simulink model "question10_2018b"  (R2018b)
settings: Solver=VariableStepAuto  StartTime=0.0  StopTime=100  RelTol=1e-3
values from neighbouring files (symbols this model uses):
  A = [ 0 1 0 0 ... (first row only)    [Alt_Industrial_plant.m]    (also in IndustrialPlant.m; ObserverExample.m = [0 1 0; 980  0  -2.8; 0 0 -100]; OldProject.m = [0 1 0 0 ;-491 0 -282.45 0; 0 0 0 1;1488 0 885.65 0]; observerWorkingExample.m = [0, 0, 1, 0)
  Ad = sys_d.a    [Alt_Industrial_plant.m]    (also in observerWorkingExample.m)
  B = [0; 1/Jd; 0; 0]    [Alt_Industrial_plant.m]    (also in IndustrialPlant.m; ObserverExample.m = [ 0; 0; 100]; OldProject.m = [0;82.33;0;-235.29]; observerWorkingExample.m = [0; 0; 1/mc; 1/(L*mc)])
  Bd = sys_d.b    [Alt_Industrial_plant.m]    (also in observerWorkingExample.m)
  Cd = sys_d.c    [Alt_Industrial_plant.m]    (also in observerWorkingExample.m)
  K = acker(A,B,des_poles)    [Alt_Industrial_plant.m]    (also in ObserverExample.m = place(A,B,[p1 p2 p3]); OldProject.m = place(A,B,Pole_fb); observerWorkingExample.m)
  K_d = acker(Ad,Bd,des_poles_d)    [Alt_Industrial_plant.m]    (also in observerWorkingExample.m)
  Ob = place(A',C,obs_poles)    [Alt_Industrial_plant.m]    (also in observerWorkingExample.m = acker(Ad',Cd',des_poles_d))
  Ob_d = acker(Ad',Cd',des_poles_d)    [Alt_Industrial_plant.m]
  Ts = 0.1    [Alt_Industrial_plant.m]    (also in observerWorkingExample.m)
  x0 = [0;15*pi/180;0;0]    [Alt_Industrial_plant.m]    (also in ObserverExample.m = [0.01 0.5 -5]; observerWorkingExample.m = [0;5*pi/180;0;0])
settings Model: Creator=Yaipiti  LastModifiedBy=Dimitri
settings DataIOCC: ReturnWorkspaceOutputs=on

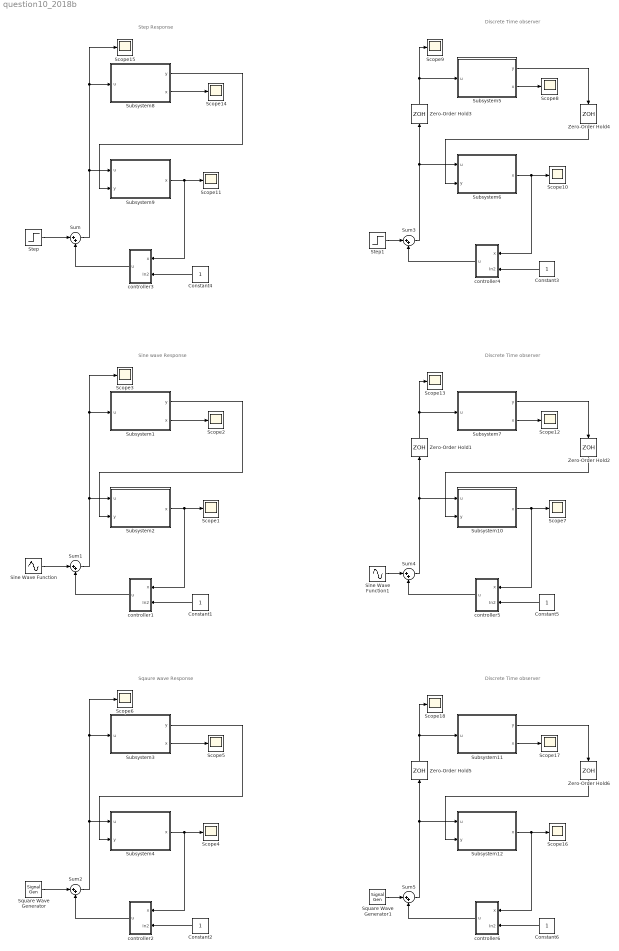
== system question10_2018b ==
  note: Step Response
  note: Sine wave Response
  note: Sqaure wave Response
  note: Discrete Time observer
  note: Discrete Time observer
  note: Discrete Time observer
  Constant{1..6} (6 alike) : Constant
  Scope{1..18} (18 alike) : Scope
  Sine Wave Function : Sin  Amplitude=2  Frequency=0.1  SampleTime=0
  Sine Wave Function1 : Sin  Amplitude=2  Frequency=0.1  SampleTime=0
  Square Wave Generator : SignalGenerator  WaveForm=square  Amplitude=5  Units=rad/sec
  Square Wave Generator1 : SignalGenerator  WaveForm=square  Amplitude=5  Units=rad/sec
  Step : Step  Time=2  SampleTime=0
  Step1 : Step  Time=2  SampleTime=0
  Subsystem1 : Subsystem
  Subsystem10 : Subsystem
  Subsystem11 : Subsystem
  Subsystem12 : Subsystem
  Subsystem2 : Subsystem
  Subsystem3 : Subsystem
  Subsystem4 : Subsystem
  Subsystem5 : Subsystem
  Subsystem6 : Subsystem
  Subsystem7 : Subsystem
  Subsystem8 : Subsystem
  Subsystem9 : Subsystem
  Sum{,1..5} (6 alike) : Sum  Inputs=|++
  Zero-Order Hold{1..6} (6 alike) : ZeroOrderHold  SampleTime=Ts
  controller1 : Subsystem
  controller2 : Subsystem
  controller3 : Subsystem
  controller4 : Subsystem
  controller5 : Subsystem
  controller6 : Subsystem
  wires:
  Constant4/1 -> controller3/2(In2)
  Subsystem8/2(x) -> Scope14/1
  Subsystem8/1(y) -> Subsystem9/2(y)
  Subsystem9/1(x) -> controller3/1(x), Scope11/1
  Step/1 -> Sum/1
  controller3/1(u) -> Sum/2
  Sum/1 -> Subsystem9/1(u), Subsystem8/1(u), Scope15/1
  controller1/1(u) -> Sum1/2
  Sine Wave Function/1 -> Sum1/1
  Subsystem2/1(x) -> controller1/1(x), Scope1/1
  Constant1/1 -> controller1/2(In2)
  Subsystem1/1(y) -> Subsystem2/2(y)
  Sum1/1 -> Subsystem2/1(u), Subsystem1/1(u), Scope3/1
  Subsystem1/2(x) -> Scope2/1
  controller2/1(u) -> Sum2/2
  Square Wave Generator/1 -> Sum2/1
  Subsystem4/1(x) -> controller2/1(x), Scope4/1
  Constant2/1 -> controller2/2(In2)
  Subsystem3/1(y) -> Subsystem4/2(y)
  Sum2/1 -> Subsystem4/1(u), Subsystem3/1(u), Scope6/1
  Subsystem3/2(x) -> Scope5/1
  Subsystem6/1(x) -> controller4/1(x), Scope10/1
  Subsystem5/2(x) -> Scope8/1
  Zero-Order Hold3/1 -> Scope9/1, Subsystem5/1(u)
  Subsystem5/1(y) -> Zero-Order Hold4/1
  Zero-Order Hold4/1 -> Subsystem6/2(y)
  Constant3/1 -> controller4/2(In2)
  Step1/1 -> Sum3/1
  controller4/1(u) -> Sum3/2
  Sum3/1 -> Subsystem6/1(u), Zero-Order Hold3/1
  Constant5/1 -> controller5/2(In2)
  Zero-Order Hold1/1 -> Scope13/1, Subsystem7/1(u)
  Zero-Order Hold2/1 -> Subsystem10/2(y)
  Subsystem7/2(x) -> Scope12/1
  Subsystem7/1(y) -> Zero-Order Hold2/1
  Sine Wave Function1/1 -> Sum4/1
  Sum4/1 -> Subsystem10/1(u), Zero-Order Hold1/1
  controller5/1(u) -> Sum4/2
  Subsystem10/1(x) -> controller5/1(x), Scope7/1
  Constant6/1 -> controller6/2(In2)
  Zero-Order Hold5/1 -> Scope18/1, Subsystem11/1(u)
  Zero-Order Hold6/1 -> Subsystem12/2(y)
  Subsystem11/2(x) -> Scope17/1
  Subsystem11/1(y) -> Zero-Order Hold6/1
  Square Wave Generator1/1 -> Sum5/1
  Sum5/1 -> Subsystem12/1(u), Zero-Order Hold5/1
  controller6/1(u) -> Sum5/2
  Subsystem12/1(x) -> controller6/1(x), Scope16/1

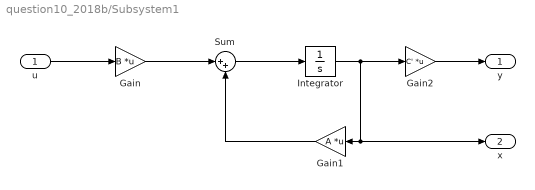
== system question10_2018b/Subsystem1 ==
  u : Inport
  Gain : Gain  Gain=B  Multiplication=Matrix(K*u)
  Gain1 : Gain  Gain=A  Multiplication=Matrix(K*u)
  Gain2 : Gain  Gain=C'  Multiplication=Matrix(K*u)
  Integrator : Integrator  InitialCondition=x0
  Sum : Sum  Inputs=|++
  y : Outport  VectorParamsAs1DForOutWhenUnconnected=on
  x : Outport  Port=2  VectorParamsAs1DForOutWhenUnconnected=on
  wires:
  Gain/1 -> Sum/1
  Sum/1 -> Integrator/1
  Gain1/1 -> Sum/2
  u/1 -> Gain/1
  Gain2/1 -> y/1
  Integrator/1 -> Gain2/1, x/1, Gain1/1

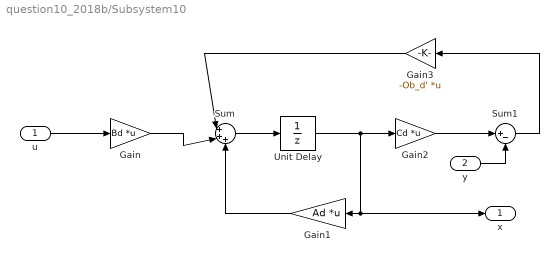
== system question10_2018b/Subsystem10 ==
  u : Inport
  y : Inport  Port=2
  Gain : Gain  Gain=Bd  Multiplication=Matrix(K*u)
  Gain1 : Gain  Gain=Ad  Multiplication=Matrix(K*u)
  Gain2 : Gain  Gain=Cd  Multiplication=Matrix(K*u)
  Gain3 : Gain  Gain=-Ob_d'  Multiplication=Matrix(K*u)
  Sum : Sum  Inputs=|+++
  Sum1 : Sum  Inputs=|+-
  Unit Delay : UnitDelay  InitialCondition=x0*0  SampleTime=-1
  x : Outport  VectorParamsAs1DForOutWhenUnconnected=on
  wires:
  u/1 -> Gain/1
  Unit Delay/1 -> Gain2/1, x/1, Gain1/1
  Sum/1 -> Unit Delay/1
  y/1 -> Sum1/2
  Gain2/1 -> Sum1/1
  Sum1/1 -> Gain3/1
  Gain1/1 -> Sum/3
  Gain/1 -> Sum/2
  Gain3/1 -> Sum/1

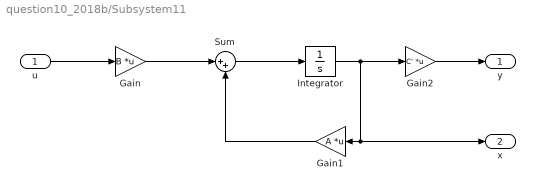
== system question10_2018b/Subsystem11 ==
  u : Inport
  Gain : Gain  Gain=B  Multiplication=Matrix(K*u)
  Gain1 : Gain  Gain=A  Multiplication=Matrix(K*u)
  Gain2 : Gain  Gain=C'  Multiplication=Matrix(K*u)
  Integrator : Integrator  InitialCondition=x0
  Sum : Sum  Inputs=|++
  y : Outport  VectorParamsAs1DForOutWhenUnconnected=on
  x : Outport  Port=2  VectorParamsAs1DForOutWhenUnconnected=on
  wires:
  Gain/1 -> Sum/1
  Sum/1 -> Integrator/1
  Gain1/1 -> Sum/2
  u/1 -> Gain/1
  Gain2/1 -> y/1
  Integrator/1 -> Gain2/1, x/1, Gain1/1

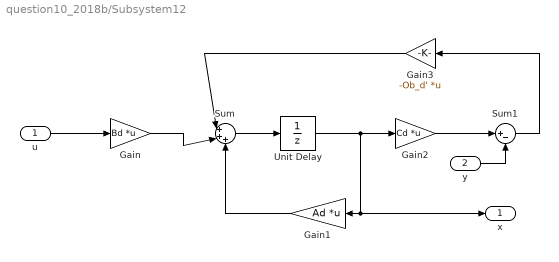
== system question10_2018b/Subsystem12 ==
  u : Inport
  y : Inport  Port=2
  Gain : Gain  Gain=Bd  Multiplication=Matrix(K*u)
  Gain1 : Gain  Gain=Ad  Multiplication=Matrix(K*u)
  Gain2 : Gain  Gain=Cd  Multiplication=Matrix(K*u)
  Gain3 : Gain  Gain=-Ob_d'  Multiplication=Matrix(K*u)
  Sum : Sum  Inputs=|+++
  Sum1 : Sum  Inputs=|+-
  Unit Delay : UnitDelay  InitialCondition=x0*0  SampleTime=-1
  x : Outport  VectorParamsAs1DForOutWhenUnconnected=on
  wires:
  u/1 -> Gain/1
  Unit Delay/1 -> Gain2/1, x/1, Gain1/1
  Sum/1 -> Unit Delay/1
  y/1 -> Sum1/2
  Gain2/1 -> Sum1/1
  Sum1/1 -> Gain3/1
  Gain1/1 -> Sum/3
  Gain/1 -> Sum/2
  Gain3/1 -> Sum/1

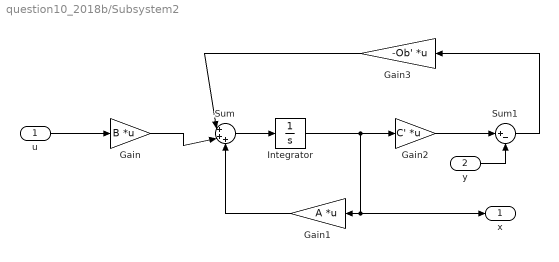
== system question10_2018b/Subsystem2 ==
  u : Inport
  y : Inport  Port=2
  Gain : Gain  Gain=B  Multiplication=Matrix(K*u)
  Gain1 : Gain  Gain=A  Multiplication=Matrix(K*u)
  Gain2 : Gain  Gain=C'  Multiplication=Matrix(K*u)
  Gain3 : Gain  Gain=-Ob'  Multiplication=Matrix(K*u)
  Integrator : Integrator
  Sum : Sum  Inputs=|+++
  Sum1 : Sum  Inputs=|+-
  x : Outport  VectorParamsAs1DForOutWhenUnconnected=on
  wires:
  u/1 -> Gain/1
  Integrator/1 -> Gain2/1, x/1, Gain1/1
  y/1 -> Sum1/2
  Gain2/1 -> Sum1/1
  Sum1/1 -> Gain3/1
  Gain1/1 -> Sum/3
  Gain/1 -> Sum/2
  Gain3/1 -> Sum/1
  Sum/1 -> Integrator/1

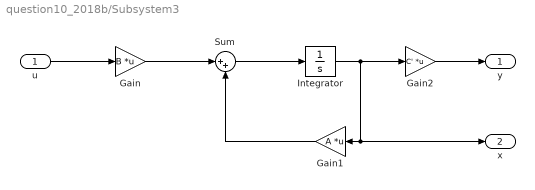
== system question10_2018b/Subsystem3 ==
  u : Inport
  Gain : Gain  Gain=B  Multiplication=Matrix(K*u)
  Gain1 : Gain  Gain=A  Multiplication=Matrix(K*u)
  Gain2 : Gain  Gain=C'  Multiplication=Matrix(K*u)
  Integrator : Integrator  InitialCondition=x0
  Sum : Sum  Inputs=|++
  y : Outport  VectorParamsAs1DForOutWhenUnconnected=on
  x : Outport  Port=2  VectorParamsAs1DForOutWhenUnconnected=on
  wires:
  Gain/1 -> Sum/1
  Sum/1 -> Integrator/1
  Gain1/1 -> Sum/2
  u/1 -> Gain/1
  Gain2/1 -> y/1
  Integrator/1 -> Gain2/1, x/1, Gain1/1

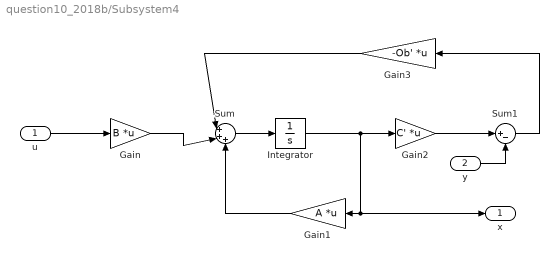
== system question10_2018b/Subsystem4 ==
  u : Inport
  y : Inport  Port=2
  Gain : Gain  Gain=B  Multiplication=Matrix(K*u)
  Gain1 : Gain  Gain=A  Multiplication=Matrix(K*u)
  Gain2 : Gain  Gain=C'  Multiplication=Matrix(K*u)
  Gain3 : Gain  Gain=-Ob'  Multiplication=Matrix(K*u)
  Integrator : Integrator
  Sum : Sum  Inputs=|+++
  Sum1 : Sum  Inputs=|+-
  x : Outport  VectorParamsAs1DForOutWhenUnconnected=on
  wires:
  u/1 -> Gain/1
  Integrator/1 -> Gain2/1, x/1, Gain1/1
  y/1 -> Sum1/2
  Gain2/1 -> Sum1/1
  Sum1/1 -> Gain3/1
  Gain1/1 -> Sum/3
  Gain/1 -> Sum/2
  Gain3/1 -> Sum/1
  Sum/1 -> Integrator/1

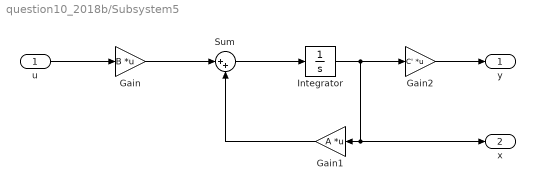
== system question10_2018b/Subsystem5 ==
  u : Inport
  Gain : Gain  Gain=B  Multiplication=Matrix(K*u)
  Gain1 : Gain  Gain=A  Multiplication=Matrix(K*u)
  Gain2 : Gain  Gain=C'  Multiplication=Matrix(K*u)
  Integrator : Integrator  InitialCondition=x0
  Sum : Sum  Inputs=|++
  y : Outport  VectorParamsAs1DForOutWhenUnconnected=on
  x : Outport  Port=2  VectorParamsAs1DForOutWhenUnconnected=on
  wires:
  Gain/1 -> Sum/1
  Sum/1 -> Integrator/1
  Gain1/1 -> Sum/2
  u/1 -> Gain/1
  Gain2/1 -> y/1
  Integrator/1 -> Gain2/1, x/1, Gain1/1

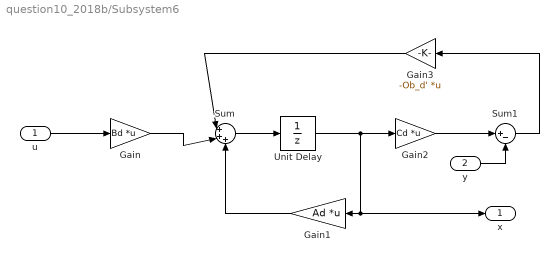
== system question10_2018b/Subsystem6 ==
  u : Inport
  y : Inport  Port=2
  Gain : Gain  Gain=Bd  Multiplication=Matrix(K*u)
  Gain1 : Gain  Gain=Ad  Multiplication=Matrix(K*u)
  Gain2 : Gain  Gain=Cd  Multiplication=Matrix(K*u)
  Gain3 : Gain  Gain=-Ob_d'  Multiplication=Matrix(K*u)
  Sum : Sum  Inputs=|+++
  Sum1 : Sum  Inputs=|+-
  Unit Delay : UnitDelay  InitialCondition=x0*0  SampleTime=-1
  x : Outport  VectorParamsAs1DForOutWhenUnconnected=on
  wires:
  u/1 -> Gain/1
  Unit Delay/1 -> Gain2/1, x/1, Gain1/1
  Sum/1 -> Unit Delay/1
  y/1 -> Sum1/2
  Gain2/1 -> Sum1/1
  Sum1/1 -> Gain3/1
  Gain1/1 -> Sum/3
  Gain/1 -> Sum/2
  Gain3/1 -> Sum/1

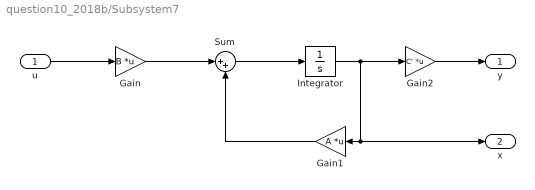
== system question10_2018b/Subsystem7 ==
  u : Inport
  Gain : Gain  Gain=B  Multiplication=Matrix(K*u)
  Gain1 : Gain  Gain=A  Multiplication=Matrix(K*u)
  Gain2 : Gain  Gain=C'  Multiplication=Matrix(K*u)
  Integrator : Integrator  InitialCondition=x0
  Sum : Sum  Inputs=|++
  y : Outport  VectorParamsAs1DForOutWhenUnconnected=on
  x : Outport  Port=2  VectorParamsAs1DForOutWhenUnconnected=on
  wires:
  Gain/1 -> Sum/1
  Sum/1 -> Integrator/1
  Gain1/1 -> Sum/2
  u/1 -> Gain/1
  Gain2/1 -> y/1
  Integrator/1 -> Gain2/1, x/1, Gain1/1

== system question10_2018b/Subsystem8 ==
  u : Inport
  Gain : Gain  Gain=B  Multiplication=Matrix(K*u)
  Gain1 : Gain  Gain=A  Multiplication=Matrix(K*u)
  Gain2 : Gain  Gain=C'  Multiplication=Matrix(K*u)
  Integrator : Integrator  InitialCondition=x0
  Sum : Sum  Inputs=|++
  y : Outport  VectorParamsAs1DForOutWhenUnconnected=on
  x : Outport  Port=2  VectorParamsAs1DForOutWhenUnconnected=on
  wires:
  Gain/1 -> Sum/1
  Sum/1 -> Integrator/1
  Gain1/1 -> Sum/2
  u/1 -> Gain/1
  Gain2/1 -> y/1
  Integrator/1 -> Gain2/1, x/1, Gain1/1

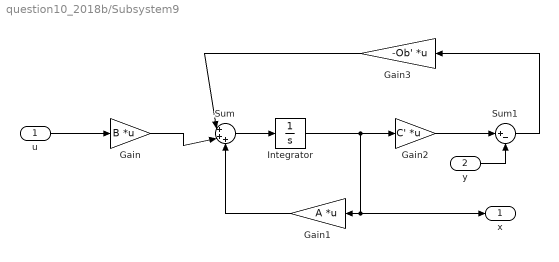
== system question10_2018b/Subsystem9 ==
  u : Inport
  y : Inport  Port=2
  Gain : Gain  Gain=B  Multiplication=Matrix(K*u)
  Gain1 : Gain  Gain=A  Multiplication=Matrix(K*u)
  Gain2 : Gain  Gain=C'  Multiplication=Matrix(K*u)
  Gain3 : Gain  Gain=-Ob'  Multiplication=Matrix(K*u)
  Integrator : Integrator
  Sum : Sum  Inputs=|+++
  Sum1 : Sum  Inputs=|+-
  x : Outport  VectorParamsAs1DForOutWhenUnconnected=on
  wires:
  u/1 -> Gain/1
  Integrator/1 -> Gain2/1, x/1, Gain1/1
  y/1 -> Sum1/2
  Gain2/1 -> Sum1/1
  Sum1/1 -> Gain3/1
  Gain1/1 -> Sum/3
  Gain/1 -> Sum/2
  Gain3/1 -> Sum/1
  Sum/1 -> Integrator/1

== system question10_2018b/controller1 ==
  x : Inport
  In2 : Inport  Port=2
  Gain : Gain  Gain=[1; 0; 0; 0]
  Gain1 : Gain  Gain=10
  Gain2 : Gain  Gain=-K  Multiplication=Matrix(K*u)
  Sum : Sum  Inputs=|+-
  u : Outport  VectorParamsAs1DForOutWhenUnconnected=on
  wires:
  Gain2/1 -> Gain1/1
  x/1 -> Sum/1
  Sum/1 -> Gain2/1
  Gain/1 -> Sum/2
  In2/1 -> Gain/1
  Gain1/1 -> u/1

== system question10_2018b/controller2 ==
  x : Inport
  In2 : Inport  Port=2
  Gain : Gain  Gain=[1; 0; 0; 0]
  Gain1 : Gain  Gain=10
  Gain2 : Gain  Gain=-K  Multiplication=Matrix(K*u)
  Sum : Sum  Inputs=|+-
  u : Outport  VectorParamsAs1DForOutWhenUnconnected=on
  wires:
  Gain2/1 -> Gain1/1
  x/1 -> Sum/1
  Sum/1 -> Gain2/1
  Gain/1 -> Sum/2
  In2/1 -> Gain/1
  Gain1/1 -> u/1

== system question10_2018b/controller3 ==
  x : Inport
  In2 : Inport  Port=2
  Gain : Gain  Gain=[1; 0; 0; 0]
  Gain1 : Gain  Gain=10
  Gain2 : Gain  Gain=-K  Multiplication=Matrix(K*u)
  Sum : Sum  Inputs=|+-
  u : Outport  VectorParamsAs1DForOutWhenUnconnected=on
  wires:
  Gain2/1 -> Gain1/1
  x/1 -> Sum/1
  Sum/1 -> Gain2/1
  Gain/1 -> Sum/2
  In2/1 -> Gain/1
  Gain1/1 -> u/1

== system question10_2018b/controller4 ==
  x : Inport
  In2 : Inport  Port=2
  Gain : Gain  Gain=[1; 0; 0; 0]
  Gain2 : Gain  Gain=-K_d  Multiplication=Matrix(K*u)
  Sum : Sum  Inputs=|+-
  u : Outport  VectorParamsAs1DForOutWhenUnconnected=on
  wires:
  Gain2/1 -> u/1
  x/1 -> Sum/1
  Sum/1 -> Gain2/1
  Gain/1 -> Sum/2
  In2/1 -> Gain/1

== system question10_2018b/controller5 ==
  x : Inport
  In2 : Inport  Port=2
  Gain : Gain  Gain=[1; 0; 0; 0]
  Gain2 : Gain  Gain=-K_d  Multiplication=Matrix(K*u)
  Sum : Sum  Inputs=|+-
  u : Outport  VectorParamsAs1DForOutWhenUnconnected=on
  wires:
  Gain2/1 -> u/1
  x/1 -> Sum/1
  Sum/1 -> Gain2/1
  Gain/1 -> Sum/2
  In2/1 -> Gain/1

== system question10_2018b/controller6 ==
  x : Inport
  In2 : Inport  Port=2
  Gain : Gain  Gain=[1; 0; 0; 0]
  Gain2 : Gain  Gain=-K_d  Multiplication=Matrix(K*u)
  Sum : Sum  Inputs=|+-
  u : Outport  VectorParamsAs1DForOutWhenUnconnected=on
  wires:
  Gain2/1 -> u/1
  x/1 -> Sum/1
  Sum/1 -> Gain2/1
  Gain/1 -> Sum/2
  In2/1 -> Gain/1
